simulink library "EmbededCommunicationModule"  (R2021a)
settings: Solver=VariableStepAuto  StartTime=0.0  StopTime=10.0  RelTol=1e-3
values from neighbouring files (symbols this model uses):
  modbus_rtu = ModbusRTU()    [InitECM.m]
settings Model: Creator=Harry  LastModifiedBy=Harry

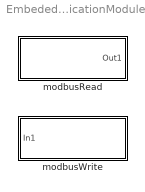
== system EmbededCommunicationModule ==
  modbusRead : Subsystem  mask{parmName='testParmName'}
      mask Display:
      | if ischar(parmName)
      |     color('black');
      |     x=sprintf('Read: %s', parmName);
      |     disp(x);
      | else
      |     color('red');
      |     disp('Input Error');
      | end
  modbusWrite : Subsystem  mask{parmName='test02'}
      mask Display:
      | if ischar(parmName)
      |     color('black');
      |     x=sprintf('Write: %s', parmName);
      |     disp(x);
      | else
      |     color('red');
      |     disp('Input Error');
      | end

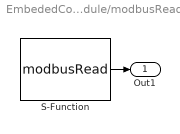
== system EmbededCommunicationModule/modbusRead ==
  S-Function : S-Function  FunctionName=modbusRead  Parameters=modbus_rtu,parmName  SFunctionDeploymentMode=off  EnableBusSupport=off
  Out1 : Outport
  wires:
  S-Function/1 -> Out1/1

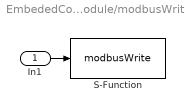
== system EmbededCommunicationModule/modbusWrite ==
  In1 : Inport
  S-Function : S-Function  FunctionName=modbusWrite  Parameters=modbus_rtu,parmName  SFunctionDeploymentMode=off  EnableBusSupport=off
  wires:
  In1/1 -> S-Function/1
